simulink model "fk"  (R2025b)
settings: Solver=VariableStepAuto  StartTime=0.0  StopTime=10.0  RelTol=1e-3
values from neighbouring files (symbols this model uses):
  q_v1 = [deg2rad(30), 100, deg2rad(-60)]    [armVars.m]
  robot = buildRobot()    [armVars.m]    (also in buildRobot.m = SerialLink(L, 'name', 'Christopher'))
libraries: roblocks x2
settings Model: Creator=leeki  LastModifiedBy=leeki

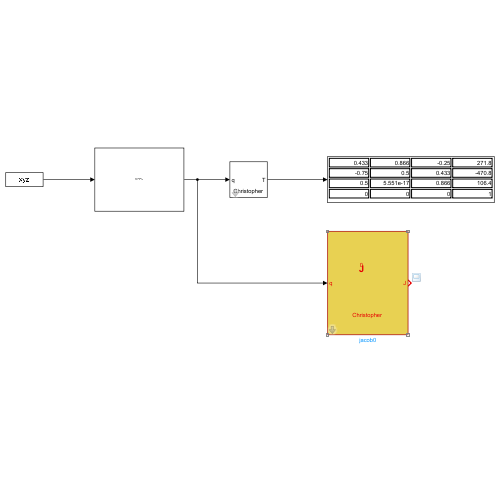
[thumbnail: Simulink's stored preview of the top-level diagram]
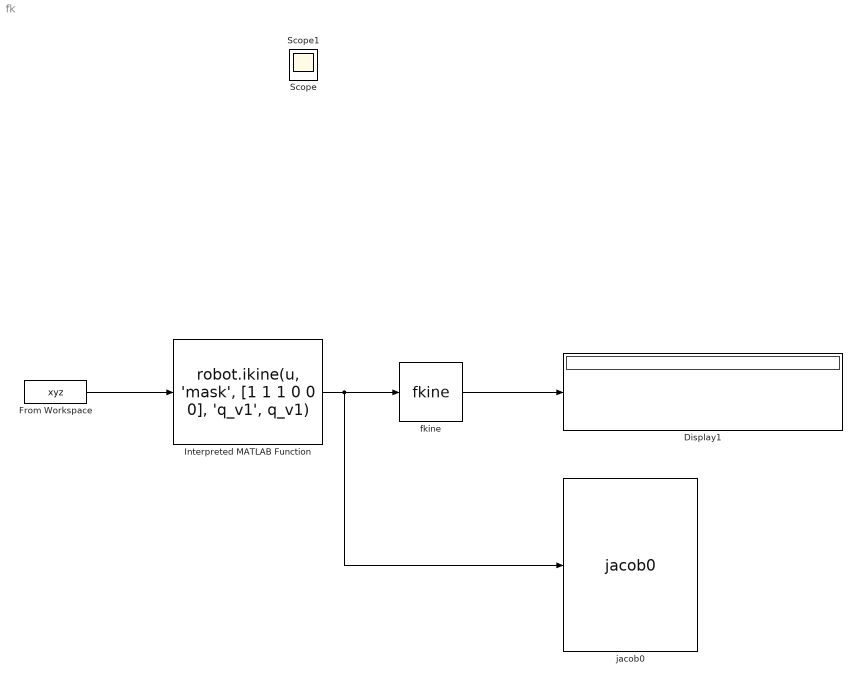
== system fk ==
  Display1 : Display
  From Workspace : FromWorkspace  VariableName=xyz  OutputAfterFinalValue=Holding final value
  Interpreted MATLAB Function : MATLABFcn  MATLABFcn=robot.ikine(u, 'mask', [1 1 1 0 0 0], 'q_v1', q_v1)  OutputDimensions=3  Output1D=off
  fkine : roblocks/Arm/fkine  robot=robot
      link override MATLAB Fcn: MATLABFcn=double(robot.fkine(u))
  "jacob0 " : roblocks/Arm/jacob0   robot=robot
      link override MATLAB Fcn: MATLABFcn=robot.jacob0(u(:)')
  Scope : Scope
  Scope1 : Scope
  wires:
  fkine/1 -> Display1/1
  From Workspace/1 -> Interpreted MATLAB Function/1
  Interpreted MATLAB Function/1 -> "jacob0 "/1, fkine/1
